simulink model "prob23"  (R2024a)
settings: Solver=VariableStepAuto  StartTime=0.0  StopTime=10  RelTol=1e-3
settings Model: Creator=Ranjeet  LastModifiedBy=Ranjeet

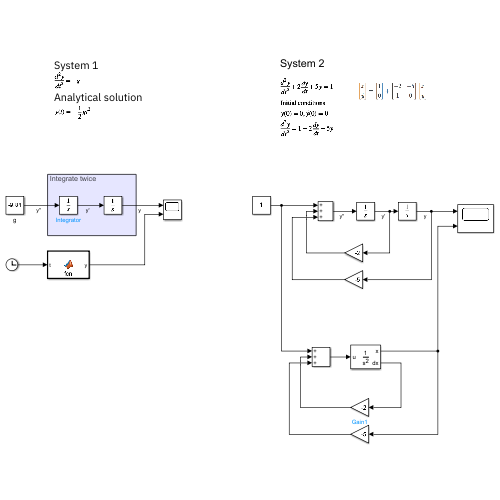
[thumbnail: Simulink's stored preview of the top-level diagram]
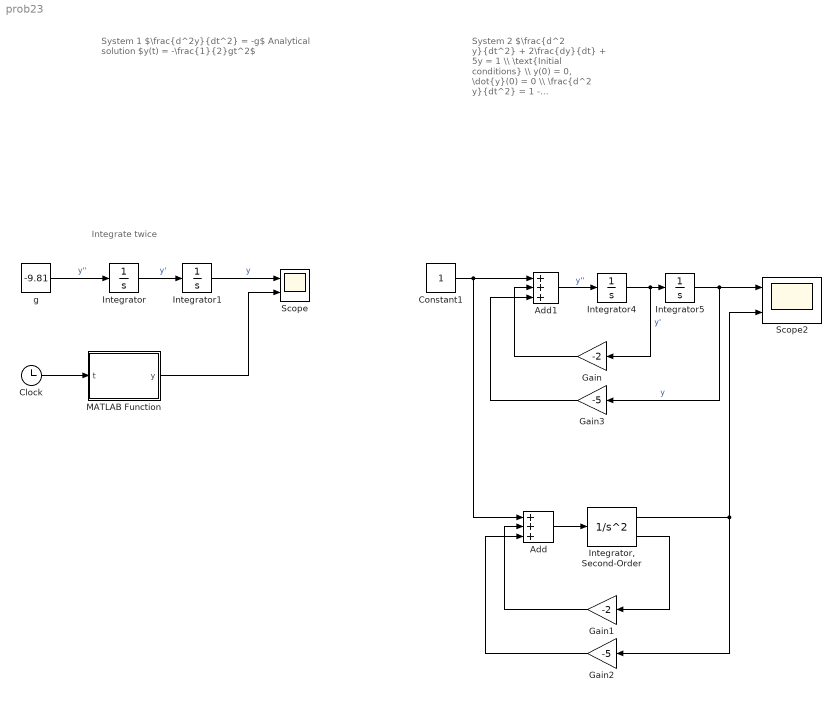
== system prob23 ==
  note: System 2
      |
      | $\frac{d^2 y}{dt^2} + 2\frac{dy}{dt} + 5y = 1 \\ \text{Initial conditions} \\ y(0) = 0, \dot{y}(0) = 0 \\ \frac{d^2 y}{dt^2} = 1 - 2\frac{dy}{dt} - 5y$
  note: Integrate twice
  note: System 1
      | $\frac{d^2y}{dt^2} = -g$
      | Analytical solution
      | $y(t) = -\frac{1}{2}gt^2$
  Add : Sum  Inputs=+++
  Add1 : Sum  Inputs=+++
  Clock : Clock
  Constant1 : Constant
  Gain : Gain  Gain=-2
  Gain1 : Gain  Gain=-2
  Gain2 : Gain  Gain=-5
  Gain3 : Gain  Gain=-5
  Integrator{,1,4..5} (4 alike) : Integrator
  "Integrator, Second-Order" : SecondOrderIntegrator
  MATLAB Function : MATLAB Function  TreatAsAtomicUnit=on
  Scope : Scope  NumInputPorts=2
  Scope2 : Scope  NumInputPorts=2
  g : Constant  Value=-9.81
  wires:
  g/1 -> Integrator/1  "y''"
  Integrator/1 -> Integrator1/1  "y'"
  Integrator1/1 -> Scope/1  "y"
  MATLAB Function/1(y) -> Scope/2
  Clock/1 -> MATLAB Function/1(t)
  Integrator4/1 -> Gain/1, Integrator5/1  "y'"
  Integrator5/1 -> Gain3/1, Scope2/1  "y"
  Add1/1 -> Integrator4/1  "y''"
  Constant1/1 -> Add/1, Add1/1
  Gain/1 -> Add1/2
  Gain3/1 -> Add1/3
  Add/1 -> "Integrator, Second-Order"/1
  "Integrator, Second-Order"/1 -> Scope2/2, Gain2/1
  "Integrator, Second-Order"/2 -> Gain1/1
  Gain1/1 -> Add/2
  Gain2/1 -> Add/3

== matlab function prob23/MATLAB Function ==
  data: t input; y output
function y = fcn(t)
g = 9.81;
y = -0.5 * g * t^2;
